simulink model "compFilter"  (Simulink 7.5)
settings: Solver=ode45  StartTime=0.0  StopTime=20  RelTol=1e-3
libraries: simulink x1
settings Model: Creator=user  LastModifiedBy=user
settings DebuggingCC: FcnCallInpInsideContextMsg=Enable All
settings GRTTargetCC: CombineOutputUpdateFcns=on

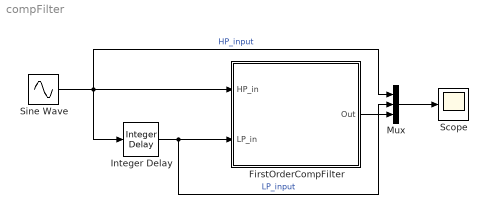
== system compFilter ==
  FirstOrderCompFilter : Subsystem
  Integer Delay : simulink/Discrete/Integer Delay  vinit=0.0  samptime=-1  NumDelays=3
  Mux : Mux  Inputs=3
  Scope : Scope
  Sine Wave : Sin  Amplitude=1  Bias=0  Frequency=0.7  Phase=0  Samples=10  SampleTime=0.1  Offset=0
  wires:
  Sine Wave/1 -> Mux/1, FirstOrderCompFilter/1(HP_in), Integer Delay/1  "HP_input"
  Integer Delay/1 -> Mux/2, FirstOrderCompFilter/2(LP_in)  "LP_input"
  FirstOrderCompFilter/1(Out) -> Mux/3
  Mux/1 -> Scope/1

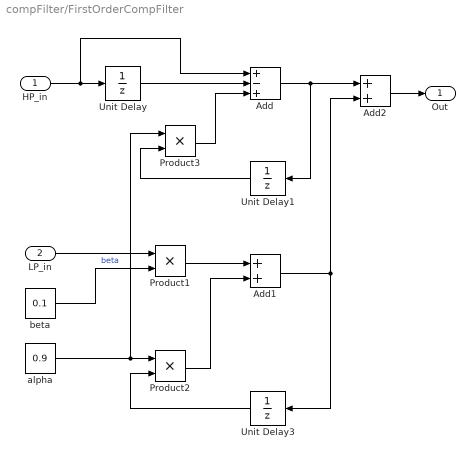
== system compFilter/FirstOrderCompFilter ==
  HP_in : Inport
  LP_in : Inport  Port=2
  Add : Sum  Inputs=+-+
  Add1 : Sum
  Add2 : Sum
  Product1 : Product  RndMeth=Zero
  Product2 : Product  RndMeth=Zero
  Product3 : Product  RndMeth=Zero
  Unit Delay : UnitDelay  SampleTime=-1
  Unit Delay1 : UnitDelay  SampleTime=-1
  Unit Delay3 : UnitDelay  SampleTime=-1
  alpha : Constant  Value=0.9
  beta : Constant  Value=0.1
  Out : Outport
  wires:
  Unit Delay/1 -> Add/2
  Add/1 -> Unit Delay1/1, Add2/1
  Add1/1 -> Unit Delay3/1, Add2/2
  Product1/1 -> Add1/1
  HP_in/1 -> Unit Delay/1, Add/1
  LP_in/1 -> Product1/1
  Add2/1 -> Out/1
  beta/1 -> Product1/2  "beta"
  alpha/1 -> Product2/1, Product3/1
  Unit Delay3/1 -> Product2/2
  Product2/1 -> Add1/2
  Product3/1 -> Add/3
  Unit Delay1/1 -> Product3/2
